simulink model "case1"  (R2024b)
settings: Solver=FixedStepAuto  StartTime=0  StopTime=1  FixedStep=1e-7  RelTol=1e-3
values from neighbouring files (symbols this model uses):
  SG_D_1_D = 0.01056    [IEEE9_case_parameters.m]    (also in case1_parameters.m; case2_parameters.m; case3_parameters.m; case4_parameters.m)
  SG_D_1_EnableSaturation = 0    [IEEE9_case_parameters.m]    (also in case1_parameters.m; case2_parameters.m; case3_parameters.m; case4_parameters.m)
  SG_D_1_f0 = 60    [IEEE9_case_parameters.m]    (also in case1_parameters.m; case2_parameters.m; case3_parameters.m; case4_parameters.m)
  SG_D_1_H = 7.5    [IEEE9_case_parameters.m]    (also in case1_parameters.m; case2_parameters.m; case3_parameters.m; case4_parameters.m)
  SG_D_1_K_A = 20    [IEEE9_case_parameters.m]    (also in case1_parameters.m; case2_parameters.m; case3_parameters.m; case4_parameters.m)
  SG_D_1_K_E = 1.000000e+1    (= 10)    [IEEE9_case_parameters.m]    (also in case1_parameters.m; case2_parameters.m; case3_parameters.m; case4_parameters.m)
  SG_D_1_K_F = 2.363    [IEEE9_case_parameters.m]    (also in case1_parameters.m; case2_parameters.m; case3_parameters.m; case4_parameters.m)
  SG_D_1_K_s = 0.5    [IEEE9_case_parameters.m]    (also in case1_parameters.m = 5; case2_parameters.m = 5; case3_parameters.m = 5; case4_parameters.m = 5)
  SG_D_1_R_a = 0.001088    [IEEE9_case_parameters.m]    (also in case1_parameters.m; case2_parameters.m; case3_parameters.m; case4_parameters.m)
  SG_D_1_S_A = 1    [IEEE9_case_parameters.m]    (also in case1_parameters.m; case2_parameters.m; case3_parameters.m; case4_parameters.m)
  SG_D_1_S_B = 0.103    [IEEE9_case_parameters.m]    (also in case1_parameters.m; case2_parameters.m; case3_parameters.m; case4_parameters.m)
  SG_D_1_S_N = 10.659857    [IEEE9_case_parameters.m]    (also in case1_parameters.m; case2_parameters.m; case3_parameters.m; case4_parameters.m)
  SG_D_1_SpeedPara = 200    [IEEE9_case_parameters.m]    (also in case1_parameters.m; case2_parameters.m; case3_parameters.m; case4_parameters.m)
  SG_D_1_T_0 = 0.720173    [IEEE9_case_parameters.m]    (also in case1_parameters.m = 0.755522; case2_parameters.m = 0.808931; case3_parameters.m = 0.869402; case4_parameters.m = 0.729316)
  SG_D_1_T_1 = 0.3    [IEEE9_case_parameters.m]    (also in case1_parameters.m; case2_parameters.m; case3_parameters.m; case4_parameters.m)
  SG_D_1_T_2 = 0.05    [IEEE9_case_parameters.m]    (also in case1_parameters.m; case2_parameters.m; case3_parameters.m; case4_parameters.m)
  SG_D_1_T_3 = 0.02    [IEEE9_case_parameters.m]    (also in case1_parameters.m; case2_parameters.m; case3_parameters.m; case4_parameters.m)
  SG_D_1_T_4 = 0.005    [IEEE9_case_parameters.m]    (also in case1_parameters.m; case2_parameters.m; case3_parameters.m; case4_parameters.m)
  SG_D_1_T_A = 0.02    [IEEE9_case_parameters.m]    (also in case1_parameters.m; case2_parameters.m; case3_parameters.m; case4_parameters.m)
  SG_D_1_T_dd = 8.000000e+0    (= 8)    [IEEE9_case_parameters.m]    (also in case1_parameters.m; case2_parameters.m; case3_parameters.m; case4_parameters.m)
  SG_D_1_T_ddd = 0.04    [IEEE9_case_parameters.m]    (also in case1_parameters.m; case2_parameters.m; case3_parameters.m; case4_parameters.m)
  SG_D_1_T_E = 0.314    [IEEE9_case_parameters.m]    (also in case1_parameters.m; case2_parameters.m; case3_parameters.m; case4_parameters.m)
  SG_D_1_T_F = 0.35    [IEEE9_case_parameters.m]    (also in case1_parameters.m; case2_parameters.m; case3_parameters.m; case4_parameters.m)
  SG_D_1_T_qd = 0.8    [IEEE9_case_parameters.m]    (also in case1_parameters.m; case2_parameters.m; case3_parameters.m; case4_parameters.m)
  SG_D_1_T_qdd = 0.02    [IEEE9_case_parameters.m]    (also in case1_parameters.m; case2_parameters.m; case3_parameters.m; case4_parameters.m)
  SG_D_1_T_speed = 0.1    [IEEE9_case_parameters.m]    (also in case1_parameters.m = 200; case2_parameters.m = 200; case3_parameters.m = 200; case4_parameters.m = 200)
  SG_D_1_T_w = 0.5    [IEEE9_case_parameters.m]    (also in case1_parameters.m; case2_parameters.m; case3_parameters.m; case4_parameters.m)
  SG_D_1_V_ref = 1.990276    [IEEE9_case_parameters.m]    (also in case1_parameters.m = 2.042296; case2_parameters.m = 2.051388; case3_parameters.m = 2.089584; case4_parameters.m = 2.01845)
  SG_D_1_w_ref = 376.991118    [IEEE9_case_parameters.m]    (also in case1_parameters.m; case2_parameters.m; case3_parameters.m; case4_parameters.m)
  SG_D_1_wb = 6.000000e+1    (= 60)    [IEEE9_case_parameters.m]    (also in case1_parameters.m; case2_parameters.m; case3_parameters.m; case4_parameters.m)
  SG_D_1_x_d = 1.9    [IEEE9_case_parameters.m]    (also in case1_parameters.m; case2_parameters.m; case3_parameters.m; case4_parameters.m)
  SG_D_1_x_dd = 0.302    [IEEE9_case_parameters.m]    (also in case1_parameters.m; case2_parameters.m; case3_parameters.m; case4_parameters.m)
  SG_D_1_x_ddd = 0.204    [IEEE9_case_parameters.m]    (also in case1_parameters.m; case2_parameters.m; case3_parameters.m; case4_parameters.m)
  SG_D_1_x_l = 0.05    [IEEE9_case_parameters.m]    (also in case1_parameters.m; case2_parameters.m; case3_parameters.m; case4_parameters.m)
  SG_D_1_x_q = 1.3    [IEEE9_case_parameters.m]    (also in case1_parameters.m; case2_parameters.m; case3_parameters.m; case4_parameters.m)
  SG_D_1_x_qd = 0.5    [IEEE9_case_parameters.m]    (also in case1_parameters.m; case2_parameters.m; case3_parameters.m; case4_parameters.m)
  SG_D_1_x_qdd = 0.3    [IEEE9_case_parameters.m]    (also in case1_parameters.m; case2_parameters.m; case3_parameters.m; case4_parameters.m)
  SG_D_2_D = 0.02    [IEEE9_case_parameters.m]    (also in case1_parameters.m; case2_parameters.m; case3_parameters.m; case4_parameters.m)
  SG_D_2_EnableSaturation = 0    [IEEE9_case_parameters.m]    (also in case1_parameters.m; case2_parameters.m; case3_parameters.m; case4_parameters.m)
  SG_D_2_f0 = 60    [IEEE9_case_parameters.m]    (also in case1_parameters.m; case2_parameters.m; case3_parameters.m; case4_parameters.m)
  SG_D_2_H = 8.000000e+0    (= 8)    [IEEE9_case_parameters.m]    (also in case1_parameters.m; case2_parameters.m; case3_parameters.m; case4_parameters.m)
  SG_D_2_K_A = 20    [IEEE9_case_parameters.m]    (also in case1_parameters.m; case2_parameters.m; case3_parameters.m; case4_parameters.m)
  SG_D_2_K_E = 1.000000e+1    (= 10)    [IEEE9_case_parameters.m]    (also in case1_parameters.m; case2_parameters.m; case3_parameters.m; case4_parameters.m)
  SG_D_2_K_F = 2.363    [IEEE9_case_parameters.m]    (also in case1_parameters.m; case2_parameters.m; case3_parameters.m; case4_parameters.m)
  SG_D_2_K_s = 0.5    [IEEE9_case_parameters.m]    (also in case1_parameters.m = 4; case2_parameters.m = 4; case3_parameters.m = 4; case4_parameters.m = 4)
  SG_D_2_R_a = 0.001088    [IEEE9_case_parameters.m]    (also in case1_parameters.m; case2_parameters.m; case3_parameters.m; case4_parameters.m)
  SG_D_2_S_A = 1    [IEEE9_case_parameters.m]    (also in case1_parameters.m; case2_parameters.m; case3_parameters.m; case4_parameters.m)
  SG_D_2_S_B = 0.103    [IEEE9_case_parameters.m]    (also in case1_parameters.m; case2_parameters.m; case3_parameters.m; case4_parameters.m)
  SG_D_2_S_N = 10.659857    [IEEE9_case_parameters.m]    (also in case1_parameters.m; case2_parameters.m; case3_parameters.m; case4_parameters.m)
  SG_D_2_SpeedPara = 200    [IEEE9_case_parameters.m]    (also in case1_parameters.m; case2_parameters.m; case3_parameters.m; case4_parameters.m)
  SG_D_2_T_0 = 1.632913    [IEEE9_case_parameters.m]    (also in case1_parameters.m = 1.632925; case2_parameters.m = 1.632915; case3_parameters.m = 1.632914; case4_parameters.m = 1.632927)
  SG_D_2_T_1 = 0.2    [IEEE9_case_parameters.m]    (also in case1_parameters.m; case2_parameters.m; case3_parameters.m; case4_parameters.m)
  SG_D_2_T_2 = 0.05    [IEEE9_case_parameters.m]    (also in case1_parameters.m; case2_parameters.m; case3_parameters.m; case4_parameters.m)
  SG_D_2_T_3 = 0.02    [IEEE9_case_parameters.m]    (also in case1_parameters.m; case2_parameters.m; case3_parameters.m; case4_parameters.m)
  SG_D_2_T_4 = 0.005    [IEEE9_case_parameters.m]    (also in case1_parameters.m; case2_parameters.m; case3_parameters.m; case4_parameters.m)
  SG_D_2_T_A = 0.02    [IEEE9_case_parameters.m]    (also in case1_parameters.m; case2_parameters.m; case3_parameters.m; case4_parameters.m)
  SG_D_2_T_dd = 7.9    [IEEE9_case_parameters.m]    (also in case1_parameters.m; case2_parameters.m; case3_parameters.m; case4_parameters.m)
  SG_D_2_T_ddd = 0.04    [IEEE9_case_parameters.m]    (also in case1_parameters.m; case2_parameters.m; case3_parameters.m; case4_parameters.m)
  SG_D_2_T_E = 0.314    [IEEE9_case_parameters.m]    (also in case1_parameters.m; case2_parameters.m; case3_parameters.m; case4_parameters.m)
  SG_D_2_T_F = 0.35    [IEEE9_case_parameters.m]    (also in case1_parameters.m; case2_parameters.m; case3_parameters.m; case4_parameters.m)
  SG_D_2_T_qd = 0.8    [IEEE9_case_parameters.m]    (also in case1_parameters.m; case2_parameters.m; case3_parameters.m; case4_parameters.m)
  SG_D_2_T_qdd = 0.015    [IEEE9_case_parameters.m]    (also in case1_parameters.m; case2_parameters.m; case3_parameters.m; case4_parameters.m)
  SG_D_2_T_speed = 0.1    [IEEE9_case_parameters.m]    (also in case1_parameters.m = 150; case2_parameters.m = 150; case3_parameters.m = 150; case4_parameters.m = 150)
  SG_D_2_T_w = 0.35    [IEEE9_case_parameters.m]    (also in case1_parameters.m; case2_parameters.m; case3_parameters.m; case4_parameters.m)
  SG_D_2_V_ref = 2.58547    [IEEE9_case_parameters.m]    (also in case1_parameters.m = 2.597896; case2_parameters.m = 2.587136; case3_parameters.m = 2.586042; case4_parameters.m = 2.599679)
  SG_D_2_w_ref = 376.991118    [IEEE9_case_parameters.m]    (also in case1_parameters.m; case2_parameters.m; case3_parameters.m; case4_parameters.m)
  SG_D_2_wb = 6.000000e+1    (= 60)    [IEEE9_case_parameters.m]    (also in case1_parameters.m; case2_parameters.m; case3_parameters.m; case4_parameters.m)
  SG_D_2_x_d = 1.8    [IEEE9_case_parameters.m]    (also in case1_parameters.m; case2_parameters.m; case3_parameters.m; case4_parameters.m)
  SG_D_2_x_dd = 0.302    [IEEE9_case_parameters.m]    (also in case1_parameters.m; case2_parameters.m; case3_parameters.m; case4_parameters.m)
  SG_D_2_x_ddd = 0.204    [IEEE9_case_parameters.m]    (also in case1_parameters.m; case2_parameters.m; case3_parameters.m; case4_parameters.m)
  SG_D_2_x_l = 0.05    [IEEE9_case_parameters.m]    (also in case1_parameters.m; case2_parameters.m; case3_parameters.m; case4_parameters.m)
  SG_D_2_x_q = 1.25    [IEEE9_case_parameters.m]    (also in case1_parameters.m; case2_parameters.m; case3_parameters.m; case4_parameters.m)
  SG_D_2_x_qd = 0.5    [IEEE9_case_parameters.m]    (also in case1_parameters.m; case2_parameters.m; case3_parameters.m; case4_parameters.m)
  SG_D_2_x_qdd = 0.3    [IEEE9_case_parameters.m]    (also in case1_parameters.m; case2_parameters.m; case3_parameters.m; case4_parameters.m)
  SG_D_3_D = 0.02    [IEEE9_case_parameters.m]    (also in case1_parameters.m; case2_parameters.m; case3_parameters.m; case4_parameters.m)
  SG_D_3_EnableSaturation = 0    [IEEE9_case_parameters.m]    (also in case1_parameters.m; case2_parameters.m; case3_parameters.m; case4_parameters.m)
  SG_D_3_f0 = 60    [IEEE9_case_parameters.m]    (also in case1_parameters.m; case2_parameters.m; case3_parameters.m; case4_parameters.m)
  SG_D_3_H = 7.7    [IEEE9_case_parameters.m]    (also in case1_parameters.m; case2_parameters.m; case3_parameters.m; case4_parameters.m)
  SG_D_3_K_A = 20    [IEEE9_case_parameters.m]    (also in case1_parameters.m; case2_parameters.m; case3_parameters.m; case4_parameters.m)
  SG_D_3_K_E = 1.000000e+1    (= 10)    [IEEE9_case_parameters.m]    (also in case1_parameters.m; case2_parameters.m; case3_parameters.m; case4_parameters.m)
  SG_D_3_K_F = 2.363    [IEEE9_case_parameters.m]    (also in case1_parameters.m; case2_parameters.m; case3_parameters.m; case4_parameters.m)
  SG_D_3_K_s = 0.2    [IEEE9_case_parameters.m]    (also in case1_parameters.m = 2; case2_parameters.m = 2; case3_parameters.m = 2; case4_parameters.m = 2)
  SG_D_3_R_a = 0.001088    [IEEE9_case_parameters.m]    (also in case1_parameters.m; case2_parameters.m; case3_parameters.m; case4_parameters.m)
  SG_D_3_S_A = 1    [IEEE9_case_parameters.m]    (also in case1_parameters.m; case2_parameters.m; case3_parameters.m; case4_parameters.m)
  SG_D_3_S_B = 0.103    [IEEE9_case_parameters.m]    (also in case1_parameters.m; case2_parameters.m; case3_parameters.m; case4_parameters.m)
  SG_D_3_S_N = 10.659857    [IEEE9_case_parameters.m]    (also in case1_parameters.m; case2_parameters.m; case3_parameters.m; case4_parameters.m)
  SG_D_3_SpeedPara = 200    [IEEE9_case_parameters.m]    (also in case1_parameters.m; case2_parameters.m; case3_parameters.m; case4_parameters.m)
  SG_D_3_T_0 = 0.850788    [IEEE9_case_parameters.m]    (also in case1_parameters.m = 0.850786; case2_parameters.m = 0.850787; case3_parameters.m; case4_parameters.m = 0.850786)
  SG_D_3_T_1 = 0.2    [IEEE9_case_parameters.m]    (also in case1_parameters.m; case2_parameters.m; case3_parameters.m; case4_parameters.m)
  SG_D_3_T_2 = 0.05    [IEEE9_case_parameters.m]    (also in case1_parameters.m; case2_parameters.m; case3_parameters.m; case4_parameters.m)
  SG_D_3_T_3 = 0.02    [IEEE9_case_parameters.m]    (also in case1_parameters.m; case2_parameters.m; case3_parameters.m; case4_parameters.m)
  SG_D_3_T_4 = 0.005    [IEEE9_case_parameters.m]    (also in case1_parameters.m; case2_parameters.m; case3_parameters.m; case4_parameters.m)
  SG_D_3_T_A = 0.02    [IEEE9_case_parameters.m]    (also in case1_parameters.m; case2_parameters.m; case3_parameters.m; case4_parameters.m)
  SG_D_3_T_dd = 8.1    [IEEE9_case_parameters.m]    (also in case1_parameters.m; case2_parameters.m; case3_parameters.m; case4_parameters.m)
  SG_D_3_T_ddd = 0.04    [IEEE9_case_parameters.m]    (also in case1_parameters.m; case2_parameters.m; case3_parameters.m; case4_parameters.m)
  SG_D_3_T_E = 0.314    [IEEE9_case_parameters.m]    (also in case1_parameters.m; case2_parameters.m; case3_parameters.m; case4_parameters.m)
  SG_D_3_T_F = 0.35    [IEEE9_case_parameters.m]    (also in case1_parameters.m; case2_parameters.m; case3_parameters.m; case4_parameters.m)
  SG_D_3_T_qd = 0.8    [IEEE9_case_parameters.m]    (also in case1_parameters.m; case2_parameters.m; case3_parameters.m; case4_parameters.m)
  SG_D_3_T_qdd = 0.015    [IEEE9_case_parameters.m]    (also in case1_parameters.m; case2_parameters.m; case3_parameters.m; case4_parameters.m)
  SG_D_3_T_speed = 0.1    [IEEE9_case_parameters.m]    (also in case1_parameters.m = 180; case2_parameters.m = 180; case3_parameters.m = 180; case4_parameters.m = 180)
  SG_D_3_T_w = 0.4    [IEEE9_case_parameters.m]    (also in case1_parameters.m; case2_parameters.m; case3_parameters.m; case4_parameters.m)
  SG_D_3_V_ref = 1.892727    [IEEE9_case_parameters.m]    (also in case1_parameters.m = 1.906439; case2_parameters.m = 1.895535; case3_parameters.m = 1.892105; case4_parameters.m = 1.906598)
  SG_D_3_w_ref = 376.991118    [IEEE9_case_parameters.m]    (also in case1_parameters.m; case2_parameters.m; case3_parameters.m; case4_parameters.m)
  SG_D_3_wb = 6.000000e+1    (= 60)    [IEEE9_case_parameters.m]    (also in case1_parameters.m; case2_parameters.m; case3_parameters.m; case4_parameters.m)
  SG_D_3_x_d = 1.85    [IEEE9_case_parameters.m]    (also in case1_parameters.m; case2_parameters.m; case3_parameters.m; case4_parameters.m)
  SG_D_3_x_dd = 0.302    [IEEE9_case_parameters.m]    (also in case1_parameters.m; case2_parameters.m; case3_parameters.m; case4_parameters.m)
  SG_D_3_x_ddd = 0.204    [IEEE9_case_parameters.m]    (also in case1_parameters.m; case2_parameters.m; case3_parameters.m; case4_parameters.m)
  SG_D_3_x_l = 0.05    [IEEE9_case_parameters.m]    (also in case1_parameters.m; case2_parameters.m; case3_parameters.m; case4_parameters.m)
  SG_D_3_x_q = 1.2    [IEEE9_case_parameters.m]    (also in case1_parameters.m; case2_parameters.m; case3_parameters.m; case4_parameters.m)
  SG_D_3_x_qd = 0.5    [IEEE9_case_parameters.m]    (also in case1_parameters.m; case2_parameters.m; case3_parameters.m; case4_parameters.m)
  SG_D_3_x_qdd = 0.3    [IEEE9_case_parameters.m]    (also in case1_parameters.m; case2_parameters.m; case3_parameters.m; case4_parameters.m)
(part 5 of 12)

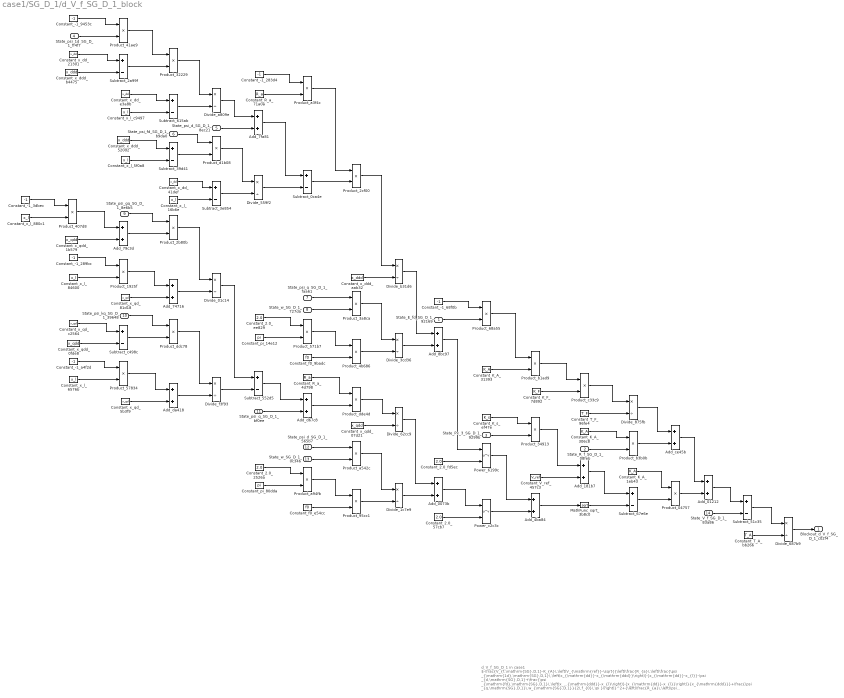
== system case1/SG_D_1/d_V_f_SG_D_1_block ==
  note: d_V_f_SG_D_1 in case1
      | $-\frac{V_{f,\mathrm{SG},D,1}-K_{A}\,\left(V_{\mathrm{ref}}-\sqrt{{\left(\frac{R_{a}\,\left(\frac{\psi _{\mathrm{1d},\mathrm{SG},D,1}\,\left(x_{\mathrm{dd}}-x_{\mathrm{ddd}}\right)}{x_{\mathrm{dd}}-x_{l}}-\psi _{d,\mathrm{SG},D,1}+\frac{\psi _{\mathrm{fd},\mathrm{SG},D,1}\,\left(x_{\mathrm{ddd}}-x_{l}\right)}{x_{\mathrm{dd}}-x_{l}}\right)}{x_{\mathrm{ddd}}}+\frac{\psi _{q,\mathrm{SG},D,1}\,w_{\mathrm{SG},D,1}}{2\,f_{0}\,\pi }\right)}^2+{\left(\frac{R_{a}\,\left(\psi _{q,\mathrm{SG},D,1}+\frac{\psi _{\mathrm{gq},\mathrm{SG},D,1}\,\left(x_{l}-x_{\mathrm{qdd}}\right)}{x_{l}-x_{\mathrm{qd}}}+\frac{\psi _{\mathrm{kq},\mathrm{SG},D,1}\,\left(x_{\mathrm{qd}}-x_{\mathrm{qdd}}\right)}{x_{l}-x_{\mathrm{qd}}}\right)}{x_{\mathrm{qdd}}}+\frac{\psi _{d,\mathrm{SG},D,1}\,w_{\mathrm{SG},D,1}}{2\,f_{0}\,\pi }\right)}^2}+K_{s}\,\mathrm{Px}_{3,\mathrm{SG},D,1}\right)-K_{A}\,R_{f,\mathrm{SG},D,1}+\frac{E_{\mathrm{fd},\mathrm{SG},D,1}\,K_{A}\,K_{F}}{T_{F}}}{T_{A}}$
      | Automatically generated on 2025-10-31 18:47:33 .
  State_E_fd_SG_D_1_92169 : Inport
  State_R_f_SG_D_1_08feb : Inport  Port=2
  State_Px_3_SG_D_1_9299b : Inport  Port=3
  State_psi_1d_SG_D_1_ff4f7 : Inport  Port=4
  State_psi_d_SG_D_1_8ec21 : Inport  Port=5
  State_psi_fd_SG_D_1_b9da0 : Inport  Port=6
  State_psi_q_SG_D_1_faa61 : Inport  Port=7
  State_w_SG_D_1_727da : Inport  Port=8
  State_psi_gq_SG_D_1_8e6b5 : Inport  Port=9
  State_psi_kq_SG_D_1_39648 : Inport  Port=10
  State_psi_q_SG_D_1_bf0ee : Inport  Port=11
  State_psi_d_SG_D_1_565b7 : Inport  Port=12
  State_w_SG_D_1_0c346 : Inport  Port=13
  State_V_f_SG_D_1_83a86 : Inport  Port=14
  Add_0073b : Sum
  Add_01212 : Sum
  Add_181b7 : Sum
  Add_4ba84 : Sum
  Add_74716 : Sum
  Add_79c3d : Sum
  Add_7fa81 : Sum
  Add_8bc97 : Sum
  Add_ce45b : Sum
  Add_d67c8 : Sum
  Add_da418 : Sum
  Constant_-1_283d4 : Constant  Value=-1
  Constant_-1_289bc : Constant  Value=-1
  Constant_-1_3dbec : Constant  Value=-1
  Constant_-1_68f0b : Constant  Value=-1
  Constant_-1_9453c : Constant  Value=-1
  Constant_-1_a4f2d : Constant  Value=-1
  Constant_2.0_2526a : Constant  Value=2.0
  Constant_2.0_57cb7 : Constant  Value=2.0
  Constant_2.0_ee829 : Constant  Value=2.0
  Constant_2.0_fd5ec : Constant  Value=2.0
  Constant_K_A_1eb43 : Constant  Value=K_A
  Constant_K_A_306c8 : Constant  Value=K_A
  Constant_K_A_31393 : Constant  Value=K_A
  Constant_K_F_7d892 : Constant  Value=K_F
  Constant_K_s_ef47e : Constant  Value=K_s
  Constant_R_a_4d798 : Constant  Value=R_a
  Constant_R_a_71a0a : Constant  Value=R_a
  Constant_T_A_bb266 : Constant  Value=T_A
  Constant_T_F_96fe4 : Constant  Value=T_F
  Constant_V_ref_457c3 : Constant  Value=V_ref
  Constant_f0_9badc : Constant  Value=f0
  Constant_f0_e54cc : Constant  Value=f0
  Constant_pi_14e12 : Constant  Value=pi
  Constant_pi_80dda : Constant  Value=pi
  Constant_x_dd_21301 : Constant  Value=x_dd
  Constant_x_dd_41def : Constant  Value=x_dd
  Constant_x_dd_e3a8b : Constant  Value=x_dd
  Constant_x_ddd_520d2 : Constant  Value=x_ddd
  Constant_x_ddd_aab32 : Constant  Value=x_ddd
  Constant_x_ddd_b4475 : Constant  Value=x_ddd
  Constant_x_l_16b6e : Constant  Value=x_l
  Constant_x_l_5f0a8 : Constant  Value=x_l
  Constant_x_l_6576b : Constant  Value=x_l
  Constant_x_l_84600 : Constant  Value=x_l
  Constant_x_l_880c1 : Constant  Value=x_l
  Constant_x_l_c9497 : Constant  Value=x_l
  Constant_x_qd_5b3f9 : Constant  Value=x_qd
  Constant_x_qd_81d18 : Constant  Value=x_qd
  Constant_x_qd_c2564 : Constant  Value=x_qd
  Constant_x_qdd_07d21 : Constant  Value=x_qdd
  Constant_x_qdd_0fde8 : Constant  Value=x_qdd
  Constant_x_qdd_1b579 : Constant  Value=x_qdd
  Divide_01c14 : Product  Inputs=*/
  Divide_1c7e9 : Product  Inputs=*/
  Divide_3cd36 : Product  Inputs=*/
  Divide_559f2 : Product  Inputs=*/
  Divide_62cc9 : Product  Inputs=*/
  Divide_687b9 : Product  Inputs=*/
  Divide_875fb : Product  Inputs=*/
  Divide_a809e : Product  Inputs=*/
  Divide_b31d6 : Product  Inputs=*/
  Divide_f3f93 : Product  Inputs=*/
  MathFunc_sqrt_3b8c0 : Sqrt
  Power_6199c : Math  Operator=pow
  Power_c2c3c : Math  Operator=pow
  Product_04757 : Product
  Product_1925f : Product
  Product_2b80b : Product
  Product_2cf00 : Product
  Product_32229 : Product
  Product_34913 : Product
  Product_3a8ca : Product
  Product_407d8 : Product
  Product_41ae9 : Product
  Product_4b686 : Product
  Product_571b7 : Product
  Product_57834 : Product
  Product_68a55 : Product
  Product_95cc1 : Product
  Product_a3f4c : Product
  Product_a542c : Product
  Product_a94fb : Product
  Product_b1ad9 : Product
  Product_b3b0b : Product
  Product_c33c9 : Product
  Product_d1b08 : Product
  Product_ddc78 : Product
  Product_dde4d : Product
  Subtract_0ca4e : Sum  Inputs=+-
  Subtract_2a99f : Sum  Inputs=+-
  Subtract_39d41 : Sum  Inputs=+-
  Subtract_3e854 : Sum  Inputs=+-
  Subtract_51c35 : Sum  Inputs=+-
  Subtract_552d5 : Sum  Inputs=+-
  Subtract_615ab : Sum  Inputs=+-
  Subtract_67e6e : Sum  Inputs=+-
  Subtract_c498c : Sum  Inputs=+-
  Blockout_d_V_f_SG_D_1_c02f4 : Outport
  wires:
  Constant_-1_a4f2d/1 -> Product_57834/1
  Constant_-1_3dbec/1 -> Product_407d8/1
  State_psi_d_SG_D_1_565b7/1 -> Product_a542c/1
  Constant_x_qd_5b3f9/1 -> Add_da418/2
  Constant_x_qdd_1b579/1 -> Add_79c3d/2
  State_w_SG_D_1_0c346/1 -> Product_a542c/2
  Constant_x_l_880c1/1 -> Product_407d8/2
  Subtract_0ca4e/1 -> Product_2cf00/2
  Constant_x_l_6576b/1 -> Product_57834/2
  Constant_x_dd_21301/1 -> Subtract_2a99f/1
  Constant_R_a_71a0a/1 -> Product_a3f4c/2
  Constant_-1_9453c/1 -> Product_41ae9/1
  Divide_559f2/1 -> Subtract_0ca4e/2
  Constant_x_ddd_b4475/1 -> Subtract_2a99f/2
  Add_da418/1 -> Divide_f3f93/2
  State_psi_1d_SG_D_1_ff4f7/1 -> Product_41ae9/2
  Add_74716/1 -> Divide_01c14/2
  Subtract_c498c/1 -> Product_ddc78/2
  Product_c33c9/1 -> Divide_875fb/1
  Product_571b7/1 -> Product_4b686/1
  Product_407d8/1 -> Add_79c3d/1
  Constant_-1_289bc/1 -> Product_1925f/1
  Constant_x_l_84600/1 -> Product_1925f/2
  Add_7fa81/1 -> Subtract_0ca4e/1
  Constant_2.0_2526a/1 -> Product_a94fb/1
  Constant_x_qd_c2564/1 -> Subtract_c498c/1
  Product_41ae9/1 -> Product_32229/1
  Constant_pi_80dda/1 -> Product_a94fb/2
  Constant_x_qdd_0fde8/1 -> Subtract_c498c/2
  Subtract_2a99f/1 -> Product_32229/2
  State_psi_q_SG_D_1_bf0ee/1 -> Add_d67c8/2
  Constant_x_dd_e3a8b/1 -> Subtract_615ab/1
  Constant_x_l_c9497/1 -> Subtract_615ab/2
  Constant_x_ddd_520d2/1 -> Subtract_39d41/1
  Constant_x_l_5f0a8/1 -> Subtract_39d41/2
  State_psi_gq_SG_D_1_8e6b5/1 -> Product_2b80b/1
  Add_79c3d/1 -> Product_2b80b/2
  Product_1925f/1 -> Add_74716/1
  Constant_x_qd_81d18/1 -> Add_74716/2
  Divide_a809e/1 -> Add_7fa81/1
  Subtract_615ab/1 -> Divide_a809e/2
  State_psi_kq_SG_D_1_39648/1 -> Product_ddc78/1
  Divide_687b9/1 -> Blockout_d_V_f_SG_D_1_c02f4/1
  Product_57834/1 -> Add_da418/1
  Product_32229/1 -> Divide_a809e/1
  State_psi_fd_SG_D_1_b9da0/1 -> Product_d1b08/1
  State_w_SG_D_1_727da/1 -> Product_3a8ca/2
  Subtract_39d41/1 -> Product_d1b08/2
  Constant_x_dd_41def/1 -> Subtract_3e854/1
  Constant_x_l_16b6e/1 -> Subtract_3e854/2
  Product_2b80b/1 -> Divide_01c14/1
  Product_a3f4c/1 -> Product_2cf00/1
  Product_ddc78/1 -> Divide_f3f93/1
  State_psi_d_SG_D_1_8ec21/1 -> Add_7fa81/2
  Product_d1b08/1 -> Divide_559f2/1
  Subtract_3e854/1 -> Divide_559f2/2
  Divide_01c14/1 -> Subtract_552d5/1
  Divide_f3f93/1 -> Subtract_552d5/2
  Constant_-1_283d4/1 -> Product_a3f4c/1
  Constant_2.0_ee829/1 -> Product_571b7/1
  Constant_pi_14e12/1 -> Product_571b7/2
  Subtract_552d5/1 -> Add_d67c8/1
  State_psi_q_SG_D_1_faa61/1 -> Product_3a8ca/1
  Constant_f0_9badc/1 -> Product_4b686/2
  Constant_R_a_4d798/1 -> Product_dde4d/1
  Add_d67c8/1 -> Product_dde4d/2
  Product_a94fb/1 -> Product_95cc1/1
  Power_6199c/1 -> Add_4ba84/1
  Constant_f0_e54cc/1 -> Product_95cc1/2
  Product_2cf00/1 -> Divide_b31d6/1
  Constant_x_ddd_aab32/1 -> Divide_b31d6/2
  Product_3a8ca/1 -> Divide_3cd36/1
  Product_4b686/1 -> Divide_3cd36/2
  Product_dde4d/1 -> Divide_62cc9/1
  Constant_x_qdd_07d21/1 -> Divide_62cc9/2
  Product_a542c/1 -> Divide_1c7e9/1
  Product_95cc1/1 -> Divide_1c7e9/2
  Divide_b31d6/1 -> Add_8bc97/1
  Divide_3cd36/1 -> Add_8bc97/2
  Divide_62cc9/1 -> Add_0073b/1
  Divide_1c7e9/1 -> Add_0073b/2
  Constant_-1_68f0b/1 -> Product_68a55/1
  State_E_fd_SG_D_1_92169/1 -> Product_68a55/2
  Add_8bc97/1 -> Power_6199c/1
  Constant_2.0_fd5ec/1 -> Power_6199c/2
  Add_0073b/1 -> Power_c2c3c/1
  Constant_2.0_57cb7/1 -> Power_c2c3c/2
  Product_68a55/1 -> Product_b1ad9/1
  Constant_K_A_31393/1 -> Product_b1ad9/2
  Constant_K_s_ef47e/1 -> Product_34913/1
  State_Px_3_SG_D_1_9299b/1 -> Product_34913/2
  Power_c2c3c/1 -> Add_4ba84/2
  Divide_875fb/1 -> Add_ce45b/1
  Product_b1ad9/1 -> Product_c33c9/1
  Constant_K_F_7d892/1 -> Product_c33c9/2
  Product_34913/1 -> Add_181b7/1
  Constant_V_ref_457c3/1 -> Add_181b7/2
  Add_4ba84/1 -> MathFunc_sqrt_3b8c0/1
  Constant_T_F_96fe4/1 -> Divide_875fb/2
  Constant_K_A_306c8/1 -> Product_b3b0b/1
  State_R_f_SG_D_1_08feb/1 -> Product_b3b0b/2
  Add_181b7/1 -> Subtract_67e6e/1
  MathFunc_sqrt_3b8c0/1 -> Subtract_67e6e/2
  Constant_T_A_bb266/1 -> Divide_687b9/2
  Product_b3b0b/1 -> Add_ce45b/2
  Constant_K_A_1eb43/1 -> Product_04757/1
  Subtract_67e6e/1 -> Product_04757/2
  Add_ce45b/1 -> Add_01212/1
  Product_04757/1 -> Add_01212/2
  Add_01212/1 -> Subtract_51c35/1
  State_V_f_SG_D_1_83a86/1 -> Subtract_51c35/2
  Subtract_51c35/1 -> Divide_687b9/1

== system case1/SG_D_1/d_psi_1d_SG_D_1_block ==
  note: d_psi_1d_SG_D_1 in case1
      | $-\frac{\psi _{\mathrm{1d},\mathrm{SG},D,1}-\psi _{\mathrm{fd},\mathrm{SG},D,1}+\frac{\left(x_{\mathrm{dd}}-x_{l}\right)\,\left(\frac{\psi _{\mathrm{1d},\mathrm{SG},D,1}\,\left(x_{\mathrm{dd}}-x_{\mathrm{ddd}}\right)}{x_{\mathrm{dd}}-x_{l}}-\psi _{d,\mathrm{SG},D,1}+\frac{\psi _{\mathrm{fd},\mathrm{SG},D,1}\,\left(x_{\mathrm{ddd}}-x_{l}\right)}{x_{\mathrm{dd}}-x_{l}}\right)}{x_{\mathrm{ddd}}}}{T_{\mathrm{ddd}}}$
      | Automatically generated on 2025-10-31 18:47:08 .
  State_psi_1d_SG_D_1_f4c7b : Inport
  State_psi_fd_SG_D_1_6f731 : Inport  Port=2
  State_psi_1d_SG_D_1_bb128 : Inport  Port=3
  State_psi_d_SG_D_1_52913 : Inport  Port=4
  State_psi_fd_SG_D_1_fd322 : Inport  Port=5
  Add_5f509 : Sum
  Add_c26bc : Sum
  Add_e5335 : Sum
  Constant_-1_7f23d : Constant  Value=-1
  Constant_-1_dee19 : Constant  Value=-1
  Constant_T_ddd_aa49e : Constant  Value=T_ddd
  Constant_x_dd_0bf0e : Constant  Value=x_dd
  Constant_x_dd_56e67 : Constant  Value=x_dd
  Constant_x_dd_ad46a : Constant  Value=x_dd
  Constant_x_dd_b4b92 : Constant  Value=x_dd
  Constant_x_ddd_4d182 : Constant  Value=x_ddd
  Constant_x_ddd_95bcc : Constant  Value=x_ddd
  Constant_x_ddd_e3c74 : Constant  Value=x_ddd
  Constant_x_l_1f274 : Constant  Value=x_l
  Constant_x_l_2cfdf : Constant  Value=x_l
  Constant_x_l_7def6 : Constant  Value=x_l
  Constant_x_l_fde22 : Constant  Value=x_l
  Divide_07f62 : Product  Inputs=*/
  Divide_0f907 : Product  Inputs=*/
  Divide_17aa0 : Product  Inputs=*/
  Divide_ccfb8 : Product  Inputs=*/
  Product_194f3 : Product
  Product_2657f : Product
  Product_46a73 : Product
  Product_6e732 : Product
  Product_7008f : Product
  Subtract_02072 : Sum  Inputs=+-
  Subtract_31294 : Sum  Inputs=+-
  Subtract_6cf4b : Sum  Inputs=+-
  Subtract_b4a13 : Sum  Inputs=+-
  Subtract_d2c18 : Sum  Inputs=+-
  Subtract_e834c : Sum  Inputs=+-
  Blockout_d_psi_1d_SG_D_1_8846c : Outport
  wires:
  Product_194f3/1 -> Product_6e732/1
  Constant_-1_dee19/1 -> Product_194f3/1
  Subtract_d2c18/1 -> Product_6e732/2
  State_psi_1d_SG_D_1_bb128/1 -> Product_194f3/2
  Subtract_31294/1 -> Product_46a73/1
  State_psi_d_SG_D_1_52913/1 -> Add_c26bc/2
  Constant_x_dd_ad46a/1 -> Subtract_02072/1
  Constant_x_l_1f274/1 -> Subtract_31294/2
  Constant_x_dd_b4b92/1 -> Subtract_d2c18/1
  Subtract_6cf4b/1 -> Product_2657f/2
  Constant_x_l_fde22/1 -> Subtract_02072/2
  Divide_0f907/1 -> Subtract_e834c/2
  Constant_x_ddd_4d182/1 -> Subtract_d2c18/2
  Constant_x_ddd_95bcc/1 -> Subtract_6cf4b/1
  Constant_x_l_2cfdf/1 -> Subtract_6cf4b/2
  Add_e5335/1 -> Add_5f509/1
  Product_6e732/1 -> Divide_17aa0/1
  Divide_ccfb8/1 -> Add_5f509/2
  Subtract_02072/1 -> Divide_17aa0/2
  State_psi_fd_SG_D_1_fd322/1 -> Product_2657f/1
  Constant_x_dd_0bf0e/1 -> Subtract_b4a13/1
  Constant_x_l_7def6/1 -> Subtract_b4a13/2
  Constant_x_ddd_e3c74/1 -> Divide_ccfb8/2
  Subtract_e834c/1 -> Product_46a73/2
  Divide_17aa0/1 -> Add_c26bc/1
  Product_2657f/1 -> Divide_0f907/1
  Subtract_b4a13/1 -> Divide_0f907/2
  Product_46a73/1 -> Divide_ccfb8/1
  Constant_x_dd_56e67/1 -> Subtract_31294/1
  Add_c26bc/1 -> Subtract_e834c/1
  Constant_-1_7f23d/1 -> Product_7008f/1
  State_psi_1d_SG_D_1_f4c7b/1 -> Product_7008f/2
  Product_7008f/1 -> Add_e5335/1
  State_psi_fd_SG_D_1_6f731/1 -> Add_e5335/2
  Add_5f509/1 -> Divide_07f62/1
  Constant_T_ddd_aa49e/1 -> Divide_07f62/2
  Divide_07f62/1 -> Blockout_d_psi_1d_SG_D_1_8846c/1

== system case1/SG_D_1/d_psi_d_SG_D_1_block ==
  note: d_psi_d_SG_D_1 in case1
      | $2\,\pi \,f_{0}\,\left(v_{d,\mathrm{SG},D,1}\,\sin\left(\theta _{\mathrm{SG},D,1}\right)-v_{q,\mathrm{SG},D,1}\,\cos\left(\theta _{\mathrm{SG},D,1}\right)+\frac{R_{a}\,\left(\frac{\psi _{\mathrm{1d},\mathrm{SG},D,1}\,\left(x_{\mathrm{dd}}-x_{\mathrm{ddd}}\right)}{x_{\mathrm{dd}}-x_{l}}-\psi _{d,\mathrm{SG},D,1}+\frac{\psi _{\mathrm{fd},\mathrm{SG},D,1}\,\left(x_{\mathrm{ddd}}-x_{l}\right)}{x_{\mathrm{dd}}-x_{l}}\right)}{x_{\mathrm{ddd}}}+\frac{\psi _{q,\mathrm{SG},D,1}\,w_{\mathrm{SG},D,1}}{2\,f_{0}\,\pi }\right)$
      | Automatically generated on 2025-10-31 18:46:44 .
  State_psi_1d_SG_D_1_5fbb9 : Inport
  State_psi_d_SG_D_1_7394f : Inport  Port=2
  State_psi_fd_SG_D_1_8eeeb : Inport  Port=3
  Input_v_d_SG_D_1_00b58 : Inport  Port=4
  State_theta_SG_D_1_4bc24 : Inport  Port=5
  Input_v_q_SG_D_1_54b58 : Inport  Port=6
  State_theta_SG_D_1_7b3a3 : Inport  Port=7
  State_psi_q_SG_D_1_4f046 : Inport  Port=8
  State_w_SG_D_1_53995 : Inport  Port=9
  Add_7f583 : Sum
  Add_f7f24 : Sum
  Constant_-1_17d18 : Constant  Value=-1
  Constant_-2.0_ae0ec : Constant  Value=-2.0
  Constant_2.0_0fc06 : Constant  Value=2.0
  Constant_R_a_82638 : Constant  Value=R_a
  Constant_f0_8f2de : Constant  Value=f0
  Constant_f0_cfcf0 : Constant  Value=f0
  Constant_pi_1f03c : Constant  Value=pi
  Constant_pi_62ad2 : Constant  Value=pi
  Constant_x_dd_1b77b : Constant  Value=x_dd
  Constant_x_dd_4aac2 : Constant  Value=x_dd
  Constant_x_dd_f0e7b : Constant  Value=x_dd
  Constant_x_ddd_8f7bc : Constant  Value=x_ddd
  Constant_x_ddd_bf976 : Constant  Value=x_ddd
  Constant_x_ddd_d3298 : Constant  Value=x_ddd
  Constant_x_l_5461b : Constant  Value=x_l
  Constant_x_l_61f70 : Constant  Value=x_l
  Constant_x_l_7559f : Constant  Value=x_l
  Divide_61754 : Product  Inputs=*/
  Divide_a0aa0 : Product  Inputs=*/
  Divide_c5597 : Product  Inputs=*/
  Divide_db4a9 : Product  Inputs=*/
  MathFunc_cos_3df25 : Trigonometry  Operator=cos
  MathFunc_sin_4e4f2 : Trigonometry
  Product_08c57 : Product
  Product_0ca52 : Product
  Product_4218c : Product
  Product_4ab49 : Product
  Product_6eda6 : Product
  Product_a3fe5 : Product
  Product_b108d : Product
  Product_b7dd3 : Product
  Product_bb5af : Product
  Product_d43e2 : Product
  Product_e2542 : Product
  Product_f75ed : Product
  Subtract_1c740 : Sum  Inputs=+-
  Subtract_3ae6e : Sum  Inputs=+-
  Subtract_43fb1 : Sum  Inputs=+-
  Subtract_5bc65 : Sum  Inputs=+-
  Subtract_6bde7 : Sum  Inputs=+-
  Subtract_ec85d : Sum  Inputs=+-
  Subtract_ee178 : Sum  Inputs=+-
  Blockout_d_psi_d_SG_D_1_c980b : Outport
  wires:
  Add_f7f24/1 -> Subtract_ec85d/1
  Product_d43e2/1 -> Divide_db4a9/1
  Subtract_43fb1/1 -> Product_d43e2/2
  Divide_db4a9/1 -> Add_f7f24/1
  Product_f75ed/1 -> Product_d43e2/1
  Constant_x_ddd_d3298/1 -> Subtract_43fb1/2
  Constant_x_dd_f0e7b/1 -> Subtract_43fb1/1
  State_psi_1d_SG_D_1_5fbb9/1 -> Product_f75ed/2
  Constant_-1_17d18/1 -> Product_f75ed/1
  Product_0ca52/1 -> Divide_a0aa0/1
  Constant_x_l_7559f/1 -> Subtract_3ae6e/2
  State_psi_d_SG_D_1_7394f/1 -> Add_f7f24/2
  Constant_x_dd_4aac2/1 -> Subtract_3ae6e/1
  Constant_x_ddd_8f7bc/1 -> Subtract_ee178/1
  Constant_x_l_61f70/1 -> Subtract_ee178/2
  Subtract_3ae6e/1 -> Divide_db4a9/2
  State_psi_fd_SG_D_1_8eeeb/1 -> Product_0ca52/1
  Constant_x_ddd_bf976/1 -> Divide_c5597/2
  Subtract_ee178/1 -> Product_0ca52/2
  Product_b108d/1 -> Subtract_5bc65/2
  Constant_x_dd_1b77b/1 -> Subtract_6bde7/1
  Constant_x_l_5461b/1 -> Subtract_6bde7/2
  Subtract_6bde7/1 -> Divide_a0aa0/2
  Divide_a0aa0/1 -> Subtract_ec85d/2
  Constant_R_a_82638/1 -> Product_e2542/1
  Subtract_ec85d/1 -> Product_e2542/2
  MathFunc_cos_3df25/1 -> Product_bb5af/2
  State_theta_SG_D_1_4bc24/1 -> MathFunc_sin_4e4f2/1
  Divide_c5597/1 -> Subtract_5bc65/1
  Product_e2542/1 -> Divide_c5597/1
  MathFunc_sin_4e4f2/1 -> Product_b108d/2
  Input_v_d_SG_D_1_00b58/1 -> Product_b108d/1
  Product_08c57/1 -> Blockout_d_psi_d_SG_D_1_c980b/1
  Product_4218c/1 -> Product_08c57/1
  Product_a3fe5/1 -> Product_4218c/1
  State_theta_SG_D_1_7b3a3/1 -> MathFunc_cos_3df25/1
  Constant_2.0_0fc06/1 -> Product_6eda6/1
  Constant_pi_62ad2/1 -> Product_6eda6/2
  Input_v_q_SG_D_1_54b58/1 -> Product_bb5af/1
  Constant_f0_cfcf0/1 -> Product_4218c/2
  State_psi_q_SG_D_1_4f046/1 -> Product_b7dd3/1
  State_w_SG_D_1_53995/1 -> Product_b7dd3/2
  Product_6eda6/1 -> Product_4ab49/1
  Constant_pi_1f03c/1 -> Product_a3fe5/2
  Constant_f0_8f2de/1 -> Product_4ab49/2
  Constant_-2.0_ae0ec/1 -> Product_a3fe5/1
  Add_7f583/1 -> Subtract_1c740/1
  Subtract_5bc65/1 -> Add_7f583/1
  Product_bb5af/1 -> Add_7f583/2
  Product_b7dd3/1 -> Divide_61754/1
  Product_4ab49/1 -> Divide_61754/2
  Divide_61754/1 -> Subtract_1c740/2
  Subtract_1c740/1 -> Product_08c57/2

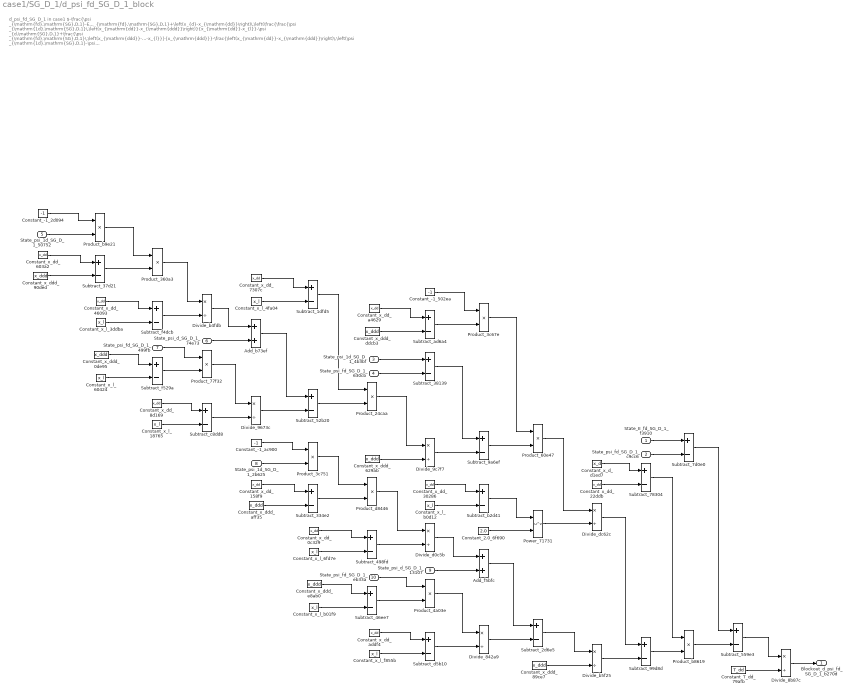
== system case1/SG_D_1/d_psi_fd_SG_D_1_block ==
  note: d_psi_fd_SG_D_1 in case1
      | $-\frac{\psi _{\mathrm{fd},\mathrm{SG},D,1}-E_{\mathrm{fd},\mathrm{SG},D,1}+\left(x_{d}-x_{\mathrm{dd}}\right)\,\left(\frac{\frac{\psi _{\mathrm{1d},\mathrm{SG},D,1}\,\left(x_{\mathrm{dd}}-x_{\mathrm{ddd}}\right)}{x_{\mathrm{dd}}-x_{l}}-\psi _{d,\mathrm{SG},D,1}+\frac{\psi _{\mathrm{fd},\mathrm{SG},D,1}\,\left(x_{\mathrm{ddd}}-x_{l}\right)}{x_{\mathrm{dd}}-x_{l}}}{x_{\mathrm{ddd}}}-\frac{\left(x_{\mathrm{dd}}-x_{\mathrm{ddd}}\right)\,\left(\psi _{\mathrm{1d},\mathrm{SG},D,1}-\psi _{\mathrm{fd},\mathrm{SG},D,1}+\frac{\left(x_{\mathrm{dd}}-x_{l}\right)\,\left(\frac{\psi _{\mathrm{1d},\mathrm{SG},D,1}\,\left(x_{\mathrm{dd}}-x_{\mathrm{ddd}}\right)}{x_{\mathrm{dd}}-x_{l}}-\psi _{d,\mathrm{SG},D,1}+\frac{\psi _{\mathrm{fd},\mathrm{SG},D,1}\,\left(x_{\mathrm{ddd}}-x_{l}\right)}{x_{\mathrm{dd}}-x_{l}}\right)}{x_{\mathrm{ddd}}}\right)}{{\left(x_{\mathrm{dd}}-x_{l}\right)}^2}\right)}{T_{\mathrm{dd}}}$
      | Automatically generated on 2025-10-31 18:47:05 .
  State_E_fd_SG_D_1_f3910 : Inport
  State_psi_fd_SG_D_1_c9cc6 : Inport  Port=2
  State_psi_1d_SG_D_1_4b3bf : Inport  Port=3
  State_psi_fd_SG_D_1_630cb : Inport  Port=4
  State_psi_1d_SG_D_1_50752 : Inport  Port=5
  State_psi_d_SG_D_1_74e73 : Inport  Port=6
  State_psi_fd_SG_D_1_499fb : Inport  Port=7
  State_psi_1d_SG_D_1_2b625 : Inport  Port=8
  State_psi_d_SG_D_1_13107 : Inport  Port=9
  State_psi_fd_SG_D_1_eb33a : Inport  Port=10
  Add_b73ef : Sum
  Add_f5bfc : Sum
  Constant_-1_2d094 : Constant  Value=-1
  Constant_-1_502ea : Constant  Value=-1
  Constant_-1_ac900 : Constant  Value=-1
  Constant_2.0_6f690 : Constant  Value=2.0
  Constant_T_dd_79afb : Constant  Value=T_dd
  Constant_x_d_d1ed7 : Constant  Value=x_d
  Constant_x_dd_0c329 : Constant  Value=x_dd
  Constant_x_dd_158f9 : Constant  Value=x_dd
  Constant_x_dd_22ddb : Constant  Value=x_dd
  Constant_x_dd_30286 : Constant  Value=x_dd
  Constant_x_dd_46093 : Constant  Value=x_dd
  Constant_x_dd_603a2 : Constant  Value=x_dd
  Constant_x_dd_7307c : Constant  Value=x_dd
  Constant_x_dd_8d169 : Constant  Value=x_dd
  Constant_x_dd_a4629 : Constant  Value=x_dd
  Constant_x_dd_addf4 : Constant  Value=x_dd
  Constant_x_ddd_0de95 : Constant  Value=x_ddd
  Constant_x_ddd_629ab : Constant  Value=x_ddd
  Constant_x_ddd_89ce7 : Constant  Value=x_ddd
  Constant_x_ddd_90ded : Constant  Value=x_ddd
  Constant_x_ddd_aff35 : Constant  Value=x_ddd
  Constant_x_ddd_ddcb3 : Constant  Value=x_ddd
  Constant_x_ddd_e8ab0 : Constant  Value=x_ddd
  Constant_x_l_18765 : Constant  Value=x_l
  Constant_x_l_3ddba : Constant  Value=x_l
  Constant_x_l_4fa04 : Constant  Value=x_l
  Constant_x_l_60424 : Constant  Value=x_l
  Constant_x_l_6fd7e : Constant  Value=x_l
  Constant_x_l_b01f9 : Constant  Value=x_l
  Constant_x_l_b0d12 : Constant  Value=x_l
  Constant_x_l_f855b : Constant  Value=x_l
  Divide_842a9 : Product  Inputs=*/
  Divide_8b87c : Product  Inputs=*/
  Divide_9673c : Product  Inputs=*/
  Divide_9c7f7 : Product  Inputs=*/
  Divide_b4fdb : Product  Inputs=*/
  Divide_b5f25 : Product  Inputs=*/
  Divide_d0c5b : Product  Inputs=*/
  Divide_dc62c : Product  Inputs=*/
  Power_71731 : Math  Operator=pow
  Product_24caa : Product
  Product_360a3 : Product
  Product_3c67e : Product
  Product_3c751 : Product
  Product_4a03e : Product
  Product_60e47 : Product
  Product_77f32 : Product
  Product_b8619 : Product
  Product_b9e21 : Product
  Product_d8446 : Product
  Subtract_1dfd5 : Sum  Inputs=+-
  Subtract_2d6e5 : Sum  Inputs=+-
  Subtract_334e2 : Sum  Inputs=+-
  Subtract_37d21 : Sum  Inputs=+-
  Subtract_38139 : Sum  Inputs=+-
  Subtract_46ee7 : Sum  Inputs=+-
  Subtract_498fd : Sum  Inputs=+-
  Subtract_52b20 : Sum  Inputs=+-
  Subtract_559e3 : Sum  Inputs=+-
  Subtract_78304 : Sum  Inputs=+-
  Subtract_7d0e0 : Sum  Inputs=+-
  Subtract_99d8d : Sum  Inputs=+-
  Subtract_9a6ef : Sum  Inputs=+-
  Subtract_ad6a4 : Sum  Inputs=+-
  Subtract_b2d41 : Sum  Inputs=+-
  Subtract_c8dd8 : Sum  Inputs=+-
  Subtract_d5b10 : Sum  Inputs=+-
  Subtract_f4dcb : Sum  Inputs=+-
  Subtract_f529a : Sum  Inputs=+-
  Blockout_d_psi_fd_SG_D_1_b270d : Outport
  wires:
  State_psi_d_SG_D_1_74e73/1 -> Add_b73ef/2
  Constant_x_dd_46093/1 -> Subtract_f4dcb/1
  Product_360a3/1 -> Divide_b4fdb/1
  Subtract_37d21/1 -> Product_360a3/2
  Subtract_52b20/1 -> Product_24caa/2
  Product_b9e21/1 -> Product_360a3/1
  Constant_x_dd_603a2/1 -> Subtract_37d21/1
  Constant_x_l_4fa04/1 -> Subtract_1dfd5/2
  Constant_-1_2d094/1 -> Product_b9e21/1
  Subtract_1dfd5/1 -> Product_24caa/1
  Constant_x_l_3ddba/1 -> Subtract_f4dcb/2
  Constant_x_ddd_90ded/1 -> Subtract_37d21/2
  State_psi_1d_SG_D_1_50752/1 -> Product_b9e21/2
  Constant_x_ddd_0de95/1 -> Subtract_f529a/1
  Constant_x_l_60424/1 -> Subtract_f529a/2
  State_E_fd_SG_D_1_f3910/1 -> Subtract_7d0e0/1
  Divide_b4fdb/1 -> Add_b73ef/1
  Subtract_f4dcb/1 -> Divide_b4fdb/2
  State_psi_fd_SG_D_1_499fb/1 -> Product_77f32/1
  Constant_x_ddd_629ab/1 -> Divide_9c7f7/2
  Subtract_f529a/1 -> Product_77f32/2
  Constant_x_dd_8d169/1 -> Subtract_c8dd8/1
  Constant_x_dd_30286/1 -> Subtract_b2d41/1
  State_psi_fd_SG_D_1_c9cc6/1 -> Subtract_7d0e0/2
  Constant_x_l_18765/1 -> Subtract_c8dd8/2
  Product_77f32/1 -> Divide_9673c/1
  Constant_-1_502ea/1 -> Product_3c67e/1
  Subtract_c8dd8/1 -> Divide_9673c/2
  Constant_x_dd_7307c/1 -> Subtract_1dfd5/1
  Add_b73ef/1 -> Subtract_52b20/1
  Constant_x_l_b0d12/1 -> Subtract_b2d41/2
  Divide_9673c/1 -> Subtract_52b20/2
  Divide_dc62c/1 -> Subtract_99d8d/1
  Constant_-1_ac900/1 -> Product_3c751/1
  State_psi_1d_SG_D_1_2b625/1 -> Product_3c751/2
  Constant_x_dd_158f9/1 -> Subtract_334e2/1
  Subtract_ad6a4/1 -> Product_3c67e/2
  Constant_x_ddd_aff35/1 -> Subtract_334e2/2
  Product_3c751/1 -> Product_d8446/1
  Constant_2.0_6f690/1 -> Power_71731/2
  Product_d8446/1 -> Divide_d0c5b/1
  Subtract_99d8d/1 -> Product_b8619/2
  Subtract_334e2/1 -> Product_d8446/2
  State_psi_d_SG_D_1_13107/1 -> Add_f5bfc/2
  Constant_x_dd_0c329/1 -> Subtract_498fd/1
  Constant_x_l_6fd7e/1 -> Subtract_498fd/2
  Constant_x_dd_a4629/1 -> Subtract_ad6a4/1
  Divide_9c7f7/1 -> Subtract_9a6ef/2
  Constant_x_ddd_e8ab0/1 -> Subtract_46ee7/1
  Constant_x_ddd_ddcb3/1 -> Subtract_ad6a4/2
  Constant_x_l_b01f9/1 -> Subtract_46ee7/2
  Subtract_46ee7/1 -> Product_4a03e/2
  State_psi_1d_SG_D_1_4b3bf/1 -> Subtract_38139/1
  Product_4a03e/1 -> Divide_842a9/1
  State_psi_fd_SG_D_1_630cb/1 -> Subtract_38139/2
  State_psi_fd_SG_D_1_eb33a/1 -> Product_4a03e/1
  Product_24caa/1 -> Divide_9c7f7/1
  Divide_d0c5b/1 -> Add_f5bfc/1
  Subtract_498fd/1 -> Divide_d0c5b/2
  Constant_x_dd_addf4/1 -> Subtract_d5b10/1
  Constant_x_l_f855b/1 -> Subtract_d5b10/2
  Divide_842a9/1 -> Subtract_2d6e5/2
  Subtract_38139/1 -> Subtract_9a6ef/1
  Subtract_d5b10/1 -> Divide_842a9/2
  Subtract_9a6ef/1 -> Product_60e47/2
  Product_3c67e/1 -> Product_60e47/1
  Subtract_b2d41/1 -> Power_71731/1
  Add_f5bfc/1 -> Subtract_2d6e5/1
  Product_60e47/1 -> Divide_dc62c/1
  Power_71731/1 -> Divide_dc62c/2
  Subtract_2d6e5/1 -> Divide_b5f25/1
  Constant_x_ddd_89ce7/1 -> Divide_b5f25/2
  Constant_x_d_d1ed7/1 -> Subtract_78304/1
  Constant_x_dd_22ddb/1 -> Subtract_78304/2
  Divide_b5f25/1 -> Subtract_99d8d/2
  Subtract_78304/1 -> Product_b8619/1
  Subtract_7d0e0/1 -> Subtract_559e3/1
  Product_b8619/1 -> Subtract_559e3/2
  Subtract_559e3/1 -> Divide_8b87c/1
  Constant_T_dd_79afb/1 -> Divide_8b87c/2
  Divide_8b87c/1 -> Blockout_d_psi_fd_SG_D_1_b270d/1

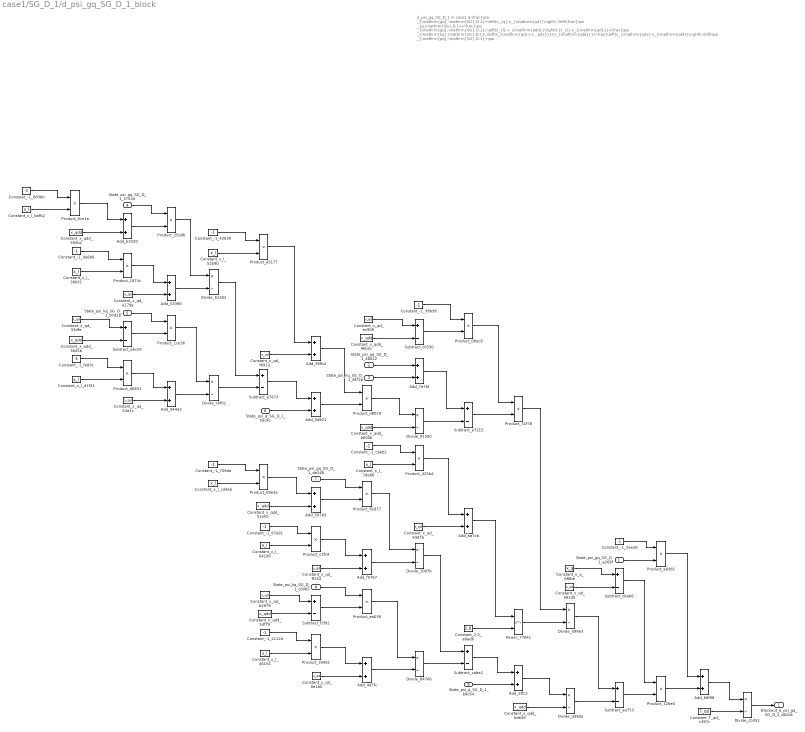
== system case1/SG_D_1/d_psi_gq_SG_D_1_block ==
  note: d_psi_gq_SG_D_1 in case1
      | $-\frac{\psi _{\mathrm{gq},\mathrm{SG},D,1}+\left(x_{q}-x_{\mathrm{qd}}\right)\,\left(\frac{\psi _{q,\mathrm{SG},D,1}+\frac{\psi _{\mathrm{gq},\mathrm{SG},D,1}\,\left(x_{l}-x_{\mathrm{qdd}}\right)}{x_{l}-x_{\mathrm{qd}}}+\frac{\psi _{\mathrm{kq},\mathrm{SG},D,1}\,\left(x_{\mathrm{qd}}-x_{\mathrm{qdd}}\right)}{x_{l}-x_{\mathrm{qd}}}}{x_{\mathrm{qdd}}}+\frac{\left(x_{\mathrm{qd}}-x_{\mathrm{qdd}}\right)\,\left(\psi _{\mathrm{gq},\mathrm{SG},D,1}+\psi _{\mathrm{kq},\mathrm{SG},D,1}+\frac{\left(x_{l}-x_{\mathrm{qd}}\right)\,\left(\psi _{q,\mathrm{SG},D,1}+\frac{\psi _{\mathrm{gq},\mathrm{SG},D,1}\,\left(x_{l}-x_{\mathrm{qdd}}\right)}{x_{l}-x_{\mathrm{qd}}}+\frac{\psi _{\mathrm{kq},\mathrm{SG},D,1}\,\left(x_{\mathrm{qd}}-x_{\mathrm{qdd}}\right)}{x_{l}-x_{\mathrm{qd}}}\right)}{x_{\mathrm{qdd}}}\right)}{{\left(x_{l}-x_{\mathrm{qd}}\right)}^2}\right)}{T_{\mathrm{qd}}}$
      | Automatically generated on 2025-10-31 18:47:12 .
  State_psi_gq_SG_D_1_a269f : Inport
  State_psi_gq_SG_D_1_48022 : Inport  Port=2
  State_psi_kq_SG_D_1_8f72b : Inport  Port=3
  State_psi_gq_SG_D_1_3753d : Inport  Port=4
  State_psi_kq_SG_D_1_97d2b : Inport  Port=5
  State_psi_q_SG_D_1_55c4c : Inport  Port=6
  State_psi_gq_SG_D_1_de248 : Inport  Port=7
  State_psi_kq_SG_D_1_c6065 : Inport  Port=8
  State_psi_q_SG_D_1_b9c64 : Inport  Port=9
  Add_044d3 : Sum
  Add_4d7fc : Sum
  Add_50783 : Sum
  Add_53390 : Sum
  Add_5d921 : Sum
  Add_66f98 : Sum
  Add_7e7bf : Sum
  Add_95fb4 : Sum
  Add_affc2 : Sum
  Add_b3320 : Sum
  Add_ba7cb : Sum
  Add_f5767 : Sum
  Constant_-1_2112d : Constant  Value=-1
  Constant_-1_2ee26 : Constant  Value=-1
  Constant_-1_38b38 : Constant  Value=-1
  Constant_-1_42039 : Constant  Value=-1
  Constant_-1_67a91 : Constant  Value=-1
  Constant_-1_683bb : Constant  Value=-1
  Constant_-1_706da : Constant  Value=-1
  Constant_-1_c9eb2 : Constant  Value=-1
  Constant_-1_da6b6 : Constant  Value=-1
  Constant_-1_fe83c : Constant  Value=-1
  Constant_2.0_a6ad6 : Constant  Value=2.0
  Constant_T_qd_c397c : Constant  Value=T_qd
  Constant_x_l_30b51 : Constant  Value=x_l
  Constant_x_l_46154 : Constant  Value=x_l
  Constant_x_l_52b9b : Constant  Value=x_l
  Constant_x_l_64199 : Constant  Value=x_l
  Constant_x_l_7de6b : Constant  Value=x_l
  Constant_x_l_bafb2 : Constant  Value=x_l
  Constant_x_l_cd4ab : Constant  Value=x_l
  Constant_x_l_d1f31 : Constant  Value=x_l
  Constant_x_q_6f6be : Constant  Value=x_q
  Constant_x_qd_0e1b0 : Constant  Value=x_qd
  Constant_x_qd_33dfe : Constant  Value=x_qd
  Constant_x_qd_53a1c : Constant  Value=x_qd
  Constant_x_qd_93d7b : Constant  Value=x_qd
  Constant_x_qd_b2879 : Constant  Value=x_qd
  Constant_x_qd_b82d5 : Constant  Value=x_qd
  Constant_x_qd_e179e : Constant  Value=x_qd
  Constant_x_qd_ec908 : Constant  Value=x_qd
  Constant_x_qd_f6913 : Constant  Value=x_qd
  Constant_x_qd_ff252 : Constant  Value=x_qd
  Constant_x_qdd_0de49 : Constant  Value=x_qdd
  Constant_x_qdd_3645b : Constant  Value=x_qdd
  Constant_x_qdd_4bb2c : Constant  Value=x_qdd
  Constant_x_qdd_51e05 : Constant  Value=x_qdd
  Constant_x_qdd_592b2 : Constant  Value=x_qdd
  Constant_x_qdd_5df79 : Constant  Value=x_qdd
  Constant_x_qdd_b000b : Constant  Value=x_qdd
  Divide_1097b : Product  Inputs=*/
  Divide_599e3 : Product  Inputs=*/
  Divide_61262 : Product  Inputs=*/
  Divide_84766 : Product  Inputs=*/
  Divide_91500 : Product  Inputs=*/
  Divide_c6f02 : Product  Inputs=*/
  Divide_cb351 : Product  Inputs=*/
  Divide_d382e : Product  Inputs=*/
  Power_77641 : Math  Operator=pow
  Product_09e3a : Product
  Product_09ec9 : Product
  Product_126e0 : Product
  Product_1874c : Product
  Product_1ce36 : Product
  Product_25ddb : Product
  Product_31f78 : Product
  Product_35461 : Product
  Product_425b4 : Product
  Product_6ce1a : Product
  Product_82d77 : Product
  Product_a8381 : Product
  Product_aa039 : Product
  Product_c3fc4 : Product
  Product_d0831 : Product
  Product_d8029 : Product
  Product_e5177 : Product
  Subtract_aa753 : Sum  Inputs=+-
  Subtract_abc59 : Sum  Inputs=+-
  Subtract_c0530 : Sum  Inputs=+-
  Subtract_cabe2 : Sum  Inputs=+-
  Subtract_dca66 : Sum  Inputs=+-
  Subtract_e7215 : Sum  Inputs=+-
  Subtract_e7673 : Sum  Inputs=+-
  Subtract_f2f92 : Sum  Inputs=+-
  Blockout_d_psi_gq_SG_D_1_d02c6 : Outport
  wires:
  State_psi_gq_SG_D_1_3753d/1 -> Product_25ddb/1
  Constant_-1_da6b6/1 -> Product_1874c/1
  Divide_61262/1 -> Subtract_e7673/1
  Add_53390/1 -> Divide_61262/2
  Product_6ce1a/1 -> Add_b3320/1
  Constant_x_qd_f6913/1 -> Add_95fb4/2
  Constant_-1_683bb/1 -> Product_6ce1a/1
  Constant_x_qdd_592b2/1 -> Add_b3320/2
  Constant_x_l_30b51/1 -> Product_1874c/2
  Constant_x_l_bafb2/1 -> Product_6ce1a/2
  Constant_-1_fe83c/1 -> Product_d0831/1
  Constant_x_qd_33dfe/1 -> Subtract_abc59/1
  Constant_x_qdd_b000b/1 -> Divide_91500/2
  Constant_x_l_d1f31/1 -> Product_d0831/2
  Constant_x_qdd_3645b/1 -> Subtract_abc59/2
  Subtract_e7673/1 -> Add_5d921/1
  Add_b3320/1 -> Product_25ddb/2
  Product_25ddb/1 -> Divide_61262/1
  Product_1874c/1 -> Add_53390/1
  Constant_x_qd_e179e/1 -> Add_53390/2
  State_psi_kq_SG_D_1_97d2b/1 -> Product_1ce36/1
  Product_d0831/1 -> Add_044d3/1
  Subtract_abc59/1 -> Product_1ce36/2
  Constant_x_qd_53a1c/1 -> Add_044d3/2
  Product_1ce36/1 -> Divide_c6f02/1
  Add_044d3/1 -> Divide_c6f02/2
  Constant_-1_38b38/1 -> Product_09ec9/1
  Constant_-1_42039/1 -> Product_e5177/1
  Add_f5767/1 -> Divide_1097b/2
  Product_35461/1 -> Add_4d7fc/1
  Subtract_f2f92/1 -> Product_aa039/2
  Constant_x_l_52b9b/1 -> Product_e5177/2
  Divide_c6f02/1 -> Subtract_e7673/2
  Subtract_dca66/1 -> Product_126e0/1
  Constant_-1_c9eb2/1 -> Product_425b4/1
  Constant_-1_706da/1 -> Product_09e3a/1
  Constant_x_l_7de6b/1 -> Product_425b4/2
  Constant_x_l_cd4ab/1 -> Product_09e3a/2
  Constant_x_qd_ff252/1 -> Add_f5767/2
  Product_e5177/1 -> Add_95fb4/1
  State_psi_q_SG_D_1_55c4c/1 -> Add_5d921/2
  Product_09e3a/1 -> Add_50783/1
  Constant_x_qdd_51e05/1 -> Add_50783/2
  Constant_-1_67a91/1 -> Product_c3fc4/1
  Constant_x_qd_0e1b0/1 -> Add_4d7fc/2
  Add_95fb4/1 -> Product_d8029/1
  Constant_x_l_64199/1 -> Product_c3fc4/2
  Constant_-1_2112d/1 -> Product_35461/1
  Constant_x_qd_b2879/1 -> Subtract_f2f92/1
  Product_d8029/1 -> Divide_91500/1
  Constant_x_l_46154/1 -> Product_35461/2
  Divide_599e3/1 -> Subtract_aa753/1
  Constant_x_qdd_5df79/1 -> Subtract_f2f92/2
  Add_5d921/1 -> Product_d8029/2
  State_psi_gq_SG_D_1_de248/1 -> Product_82d77/1
  Add_50783/1 -> Product_82d77/2
  Product_c3fc4/1 -> Add_f5767/1
  State_psi_kq_SG_D_1_c6065/1 -> Product_aa039/1
  Add_4d7fc/1 -> Divide_84766/2
  State_psi_gq_SG_D_1_48022/1 -> Add_7e7bf/1
  Constant_x_qd_ec908/1 -> Subtract_c0530/1
  Constant_x_qdd_4bb2c/1 -> Subtract_c0530/2
  Product_aa039/1 -> Divide_84766/1
  State_psi_kq_SG_D_1_8f72b/1 -> Add_7e7bf/2
  Product_82d77/1 -> Divide_1097b/1
  Subtract_c0530/1 -> Product_09ec9/2
  Add_7e7bf/1 -> Subtract_e7215/1
  Divide_91500/1 -> Subtract_e7215/2
  Product_425b4/1 -> Add_ba7cb/1
  Constant_x_qd_93d7b/1 -> Add_ba7cb/2
  Divide_1097b/1 -> Subtract_cabe2/1
  Divide_84766/1 -> Subtract_cabe2/2
  Product_09ec9/1 -> Product_31f78/1
  Subtract_e7215/1 -> Product_31f78/2
  Add_ba7cb/1 -> Power_77641/1
  Constant_2.0_a6ad6/1 -> Power_77641/2
  Subtract_cabe2/1 -> Add_affc2/1
  State_psi_q_SG_D_1_b9c64/1 -> Add_affc2/2
  Product_31f78/1 -> Divide_599e3/1
  Power_77641/1 -> Divide_599e3/2
  Add_affc2/1 -> Divide_d382e/1
  Constant_x_qdd_0de49/1 -> Divide_d382e/2
  Constant_x_q_6f6be/1 -> Subtract_dca66/1
  Constant_x_qd_b82d5/1 -> Subtract_dca66/2
  Divide_d382e/1 -> Subtract_aa753/2
  Constant_-1_2ee26/1 -> Product_a8381/1
  State_psi_gq_SG_D_1_a269f/1 -> Product_a8381/2
  Subtract_aa753/1 -> Product_126e0/2
  Product_a8381/1 -> Add_66f98/1
  Product_126e0/1 -> Add_66f98/2
  Add_66f98/1 -> Divide_cb351/1
  Constant_T_qd_c397c/1 -> Divide_cb351/2
  Divide_cb351/1 -> Blockout_d_psi_gq_SG_D_1_d02c6/1
